simulink model "SixDOFSim"  (R2020b)
settings: Solver=VariableStepAuto  StartTime=0.0  StopTime=80  RelTol=1e-3
values from neighbouring files (symbols this model uses):
  A = sys_ol.A    [cost_condition_number.m]    (also in cost_coupling_control.m; cost_filter.m; coupling_control_scratch.m = sys.A; coupling_control_scratch2.m = sys.A)
  B = sys_ol.B    [cost_condition_number.m]    (also in cost_coupling_control.m; cost_filter.m; coupling_control_scratch.m = sys.B; coupling_control_scratch2.m = sys.B)
  C_tilde = zeros(size(C,1), size(A,1))    [SixDOFModel.m]    (also in cost_condition_number.m = struct_cond.C_tilde; cost_coupling_control.m = struct_cond.C_tilde; cost_filter.m = struct_cond.C_tilde; coupling_controller.m = T*C_resort)
  deltaX_init = Tx\deltaX_init    [SixDOFModel.m]    (also in coupling_controller_main.m = X_init-X_ap_simulink)
  eta_max = 15*pi/180    (= 0.261799387799)    [SixDOFModel.m]    (also in coupling_controller_main.m = 0.174532925199; load_messung_one_massmodel.m = 0.174532925199)
  eta_min = - 30*pi/180    (= -0.523598775598)    [SixDOFModel.m]    (also in coupling_controller_main.m = -0.436332312999; load_messung_one_massmodel.m = -0.436332312999)
  F = real(F)    [coupling_control_scratch.m]    (also in coupling_control_scratch2.m; coupling_controller.m = Kopt{end}; coupling_controller_main.m = -inv(C*(Ak\B)); coupling_controller_philipp.m = -inv(C*(Ak\B)))
  F_mod = F_ent(:,1:p/2)    [SixDOFModel.m]    (also in coupling_controller_main.m = F1*Q_mod; coupling_controller_philipp.m = F1*Q_mod; script_kein_theta_verk.m = F1*Q_mod)
  K_coupling = inv(Dstar)*compR    [SixDOFModel.m]    (also in coupling_controller_main.m = Kopt{1}; coupling_controller_philipp.m = Kopt{1}; script_kein_theta_verk.m = Kopt{1})
  latlon_init = [0;0]    [SixDOFModel.m]    (also in create_multi_model.m)
  m = i-1    [coupling_control_scratch.m]    (also in coupling_control_scratch2.m; defineABC.m = size(B_1,2) + size(B_2,2); implicit_linmod.m = length(U_ap); initializeParameters.m = 120000)
  noise_weight = [10 10 10 1 1 1 1 1 10 10 10 10 1 1 1 1 1 10]'    [SixDOFModel.m]
  P_e_init_1 = [0;0;-h_init_1]    [SixDOFModel.m]    (also in create_multi_model.m)
  P_e_init_2 = [0;0;-h_init_2]    [SixDOFModel.m]    (also in create_multi_model.m)
  q = X(5)    [nonlinear_6DOF.m]    (also in normieren.m = size (C,1))
  r = 5    [coupling_controller.m]    (also in coupling_controller_main.m = 100; coupling_controller_philipp.m = 200; nonlinear_6DOF.m = X(6); polgebiet.m = a2)
  sigmaf_max = 20*pi/180    (= 0.349065850399)    [SixDOFModel.m]    (also in coupling_controller_main.m; load_messung_one_massmodel.m)
  sigmaf_min = 0.5*pi/180    (= 0.00872664625997)    [SixDOFModel.m]    (also in coupling_controller_main.m; load_messung_one_massmodel.m)
  Tu = eye(size(B,2))    [SixDOFModel.m]    (also in normieren.m = zeros(p,p))
  Tx = eye(n)    [SixDOFModel.m]    (also in normieren.m = diag([200 15 50 0.1 0.1 0.1 45*pi/180 45*pi/180 10000 200 15)
  Ty = eye(size(C,1))    [SixDOFModel.m]    (also in normieren.m = zeros(q,q))
  U_ap = Tu\U_ap    [SixDOFModel.m]    (also in coupling_controller_main.m = AP(1,1).U_ap; create_multi_model.m = [U_ap_1;U_ap_2]; fsolve_trim.m = ap(11:14); trimValues.m = Z_ap(11:14))
  W_ap = W_ap(1:4)    [SixDOFModel.m]    (also in coupling_controller_philipp.m = (C*X_ap_simulink)')
  X_ap = [X_ap_1;X_ap_2]    [SixDOFModel.m]    (also in coupling_controller_main.m = AP(1,1).X_ap; create_multi_model.m; fsolve_trim.m = ap(1:10); trimValues.m = Z_ap(1:10))
  X_ap_simulink = Tx\X_ap_simulink    [SixDOFModel.m]    (also in coupling_controller_main.m = AP(1,1).X_ap_simulink; create_multi_model.m = [X_ap(1:8);X_ap(10);X_ap(11:18);X_ap(20)])
  X_init = Tx\X_init    [SixDOFModel.m]    (also in cost_coupling_control.m = struct_cond.X_init; cost_filter.m = struct_cond.X_init; coupling_controller_main.m = X_ap_simulink; create_multi_model.m = [X_init_1; X_init_2])
  xi_max = 25*pi/180    (= 0.436332312999)    [SixDOFModel.m]    (also in coupling_controller_main.m; load_messung_one_massmodel.m)
  xi_min = - xi_max    (= -0.436332312999)    [SixDOFModel.m]    (also in coupling_controller_main.m; load_messung_one_massmodel.m)
  zita_max = 30*pi/180    (= 0.523598775598)    [SixDOFModel.m]    (also in coupling_controller_main.m; load_messung_one_massmodel.m)
  zita_min = - zita_max    (= -0.523598775598)    [SixDOFModel.m]    (also in coupling_controller_main.m; load_messung_one_massmodel.m)
undefined symbols (not defined in the file or in its folder): Earth, globalParameters, Light, MIL, WGS84
libraries: aerolibfltsims x24, aerolibtransform2 x4, aerolibwind2 x4, simulink x3, shared6dof x1, aerolibanim x1
(part 3 of 3)

== matlab function SixDOFSim/6 DOF Non Linear Model Equations/MATLAB Function1 ==
  data: X input; dX output; U input; psi input; plane_selector input
function dX  = nonlinear_equations_simulink(X,U,psi,plane_selector)
%--------------States------------%
u = X(1);
v = X(2);
w = X(3);
p = X(4);
q = X(5);
r = X(6);
phi = X(7);
theta = X(8);
h = X(9);

%--------------Control------------%
eta = U(1);
sigmaf = U(2);
xi = U(3);
zita = U(4);

%--------------Constants------------%
%% Initialize
g = 9.81; %Gravity [m/s^2]
m = 120000; %Mass [kg]

%Refuel
m_fuel = 28000; %Mass of the fuel
time_refuel = 20; % Time to refuel in sec
start_time_refuel = 10; 
refuel = 0; %Without refuel = 1, with refuel = 0

% Modelling the atmosphere 
rho_const = 1.225; %Airdensity (simplification)
omega_e = 7.29211510*10^(-5); %Rotation Speed of earth [rad/s]
%omega_e = 0;
he = 6356752; %Earth radius [m]
Omega_e_tilde = vecToMat([0;0;omega_e]);

% Inertia and Paramethers of the plane
S = 260; % Flugfläche (wing platform area)
St = 64; %Aerea of the Tail [m^2] 
lt = 24.8; %Length to tail [m] (estimation)
l = 6.6; % generalized length [m]

%Moments of Inertia of Boeing 757-200 [kg(m^2]
% Ix = 10710000; % 
% Ixz = 0; 
% Iy = 14883800; 
% Iz = 25283271; 
% I = [Ix 0 Ixz;0 Iy 0;Ixz 0 Iz]; %Trägheitstensor
I = m*[40.07 0 2.09;0 64 0;2.09 0 99.92];
I_inv = inv(I);

b = 44.8; %Span [m] 
c = 6.6; % Wing Chord [m]

%Aerodynamical Positions
% P_centerGravity = [0.23*c;0;0];
% P_aerodynCenter = [0.12*c;0;0];
P_centerGravity = [0;0;0];
P_aerodynCenter = P_centerGravity;

%Motor and Thrust
%P_thrust = [0.23*c;0;0.1*c+1.9]; %Position of the motor [m] 
P_thrust = [0;0;1.9]; %Position of the motor [m] 
% P_thrust = P_centerGravity;
i_f = 0 ; %Direction of Thrus [rad];
F_max = m*g; %Warning - This is obviusly not the max thrust produced by the turbines. The max Turbine Force is considered on the maximum value of sigmaf

globalParameters.g = g;
globalParameters.m = m;
globalParameters.Omega_e_tilde = Omega_e_tilde;
globalParameters.rho_const = rho_const;
globalParameters.I = I;
globalParameters.I_inv = I_inv;
globalParameters.S = S;
globalParameters.St = St;
globalParameters.lt = lt;
globalParameters.b = b;
globalParameters.c = c;
globalParameters.l = l;
globalParameters.P_thrust =P_thrust;
globalParameters.P_centerGravity = P_centerGravity;
globalParameters.P_aerodynCenter = P_aerodynCenter;
globalParameters.i_f =i_f;
globalParameters.Fmax = F_max;
globalParameters.m_fuel = m_fuel;
globalParameters.time_refuel = time_refuel;
globalParameters.start_time_refuel = start_time_refuel;
globalParameters.refuel = refuel;

%%
T   = 288.15 - 0.0065*h;                    % Temperatur bei H
ps  = 101325*(T/288.15)^(g/1.86584);        % Statischer Luftdruck
rho = ps/(287.053*T);
if plane_selector == 1
    I = globalParameters.I ;
    S = globalParameters.S ;
    St = globalParameters.St ;
    lt = globalParameters.lt ;
    b = globalParameters.b ;
    c = globalParameters.c ;
    P_thrust = globalParameters.P_thrust ;
    P_centerGravity = globalParameters.P_centerGravity ;
    P_aerodynCenter = globalParameters.P_aerodynCenter ;
    i_f = globalParameters.i_f ;
    F_max = globalParameters.Fmax;
elseif plane_selector == 2
    I = globalParameters.I ;
    S = globalParameters.S ;
    St = globalParameters.St ;
    lt = globalParameters.lt ;
    b = globalParameters.b ;
    c = globalParameters.c ;
    P_thrust = globalParameters.P_thrust ;
    P_centerGravity = globalParameters.P_centerGravity ;
    P_aerodynCenter = globalParameters.P_aerodynCenter ;
    i_f = globalParameters.i_f ;
    F_max = globalParameters.Fmax;
end
    
% Airdynamical Coefficients
%CA0 = 1.104;
grad_alpha = 5.5;
alpha_L0 = -11.5*pi/180;
gradient_alpha_epsolon = 0.25;
gradient_CQ_Cbeta = -1.6;
gradientCQ_Czita = 0.24;
CW0 = 0.13;
kappa = 0.07;

% %--------------Variables------------%
% u = sqrt(vA^2*(1-sin(beta)^2)/(1+tan(alpha)^2));
% v = sin(beta)*vA;
% w = u*tan(alpha);
V = [u;v;w];
vA = sqrt(u^2+v^2+w^2);
alpha = atan(w/u);
beta = asin(v/vA);
gamma = theta - alpha;
dh = vA*sin(gamma);

q_d = 0.5*rho*vA^2; %Dynamic Preassure
Omega = [p;q;r];


%--------------Aerodynamical Coefficients------------%
%Forces Coefficients
CA_F = grad_alpha*(alpha - alpha_L0);
epsolon = gradient_alpha_epsolon*(alpha - alpha_L0); %Downwash [rad]
alpha_t = alpha - epsolon + eta +1.3*q*lt/vA; %Angle of Attack of the Tail [rad]
CA_H = 3.1*(St/S)*alpha_t; %Lift Coefficient of the Control Aereas (Elevator-Tail)
CA = CA_F + CA_H; %Total Lift Coefficient

CW = CW0 + kappa*(CA_F - 0.45)^2; %Drag Coefficient

CQ = gradient_CQ_Cbeta*beta + gradientCQ_Czita*zita; % Sideforce coefficient

%Moments Coefficients
N = [-1.4*beta;-0.59-3.1*(St*lt/(l*S))*(alpha-epsolon);(1-alpha*(180/(15*pi)))*beta]; %Static Moments Effects
Jakobi_CM_X = (l/vA)*[-11,    0,           5;
                      0,-4.03*St*lt^2/(S*l^2),0;
                      1.7,          0   , -11.5];
Jakobi_CM_U = [-0.6, 0, 0.22;
               0,    -3.1*St*lt/(S*l),0;
               0, 0, -0.63];      % Dependence of Control Variables
           
C_torque = N + Jakobi_CM_X*Omega + Jakobi_CM_U*[xi;eta;zita];
CL = C_torque(1);
CM = C_torque(2);
CN = C_torque(3);

%-------------- Forces and Moments ------------%
%Aerodynamics
A = q_d*S*CA; %Lift Force [N]
W = q_d*S*CW; %Air Resistance [N]
Q = q_d*S*CQ; %Transverse Force [N]

% EVTL VORZEICHEN VON BETA ÄNDERN
Tfa = coordTransfMatrix(alpha,2)*coordTransfMatrix(-beta,3); %Transformation Matrix Aerodynamics -> Körperfest

RA_a =[-W;Q;-A]; %Aerodynamical Force in Aerdodynamical Reference Frame
RA = Tfa*RA_a; %Aerodynamical Force in Body Reference Frame
QA_aerodynCenter = q_d*S*[b*CL*0.5;c*CM;b*CN*0.5]; %Torque on the aerodynamical Center
QA = QA_aerodynCenter + vecToMat(P_centerGravity- P_aerodynCenter)*RA; %Aerodynamical Force in Body Reference Frame


%Thrust
F_res = F_max*sigmaf; %Thrust Force Absolute Value
Rf = F_res*[cos(i_f);0;sin(i_f)]; %Thrust Force 
Qf = vecToMat(P_thrust - P_centerGravity)*Rf; %Thrust Moment

Q_total = Qf + QA; %Sum of external Moments in Body reference Frame [Nm]
R_total = RA + Rf; %Sum of external Forces in Body reference Frame [N]

%-------------- Equations of Motion ------------%
%Dynamic
Tfg =  coordTransfMatrix(phi,1)*coordTransfMatrix(theta,2)*coordTransfMatrix(psi,3); % Transformation Matrix goedetic --> body reference Frame
Tgf = Tfg.';%Transformation to North East Down
Omega_tilde = vecToMat(Omega);
dOmega = I_inv*(Q_total - Omega_tilde*I*Omega); %Derivative of Rotation Rate (body Reference Frame)

% ACHTUNG: Omega_e_tilde wurde in DGL für dV entfernt, da flache ERde
dV = R_total/m + Tfg*[0;0;g] - (Omega_tilde)*V; %Derivatitive of the Speed (body Reference Frame)
% dvA = (u*dV(1) + v*dV(2) + w*dV(3))/sqrt(u^2 + v^2 + w^2); %Derivative of the Approach Speed
% dalpha = (dV(3)*u - dV(1)*w)/(u^2 + u*w); %Derivative of Angle of Attack
% dbeta = (dV(2)*vA - dvA*V(2))/(vA*sqrt(vA^2 - V(2)^2)); %Derivative of Sideslip Angle

%Kinematics
dP_e = Tgf*V; % gilt nur für z-Komponente

% ACHTUNG: dh anders als im Buch ... Teg fehlt, sollte für dh keinen
% Unterschied machen
% dh = - dP_e(3); %Derivative of z-position (earth Reference Frame)

J = 1/cos(theta)*[cos(theta) sin(phi)*sin(theta) cos(phi)*sin(theta) ;0 cos(phi)*cos(theta) -sin(phi)*cos(theta);0 sin(phi) cos(phi)]; %Rotation rate matrix
dPhi = J*Omega; %Derivative of Euler Angles
dX = double([dV;dOmega;dPhi(1);dPhi(2);dh]);
end

== matlab function SixDOFSim/6 DOF Non Linear Model Equations/calc dpsi ==
  data: X input; dpsi output
function dpsi = fcn(X)
q = X(5);
r = X(6);
phi = X(7);
theta = X(8);
dpsi = (r*cos(phi))/cos(theta) + (q*sin(phi))/cos(theta);
end

== matlab function SixDOFSim/6 DOF Non Linear Model Equations/calc dpsi1 ==
  data: X input; dpsi output
function dpsi = fcn(X)
q = X(5);
r = X(6);
phi = X(7);
theta = X(8);
dpsi = (r*cos(phi))/cos(theta) + (q*sin(phi))/cos(theta);
end

== matlab function SixDOFSim/6 DOF Non Linear Model Equations/MATLAB Function2 ==
  data: X input; y output
function y = fcn(X)
u = X(1);
w = X(3);
theta = X(8);
y = theta - atan(w/u);
end

== matlab function SixDOFSim/6 DOF Model Boeing 757 200/MATLAB Function3 ==
  data: Phi input; DCM output
function DCM = getTfg(Phi)

DCM = coordTransfMatrix(Phi(1),1)*coordTransfMatrix(Phi(2),2)*coordTransfMatrix(Phi(3),3); % Transformation Matrix goedetic --> body reference Frame

== matlab function SixDOFSim/6 DOF Model Boeing 757 200/Rho/calc_rho ==
  data: h input; rho output; globalParameters parameter
function rho = fcn(h,globalParameters)
g = globalParameters.g;
T   = 288.15 - 0.0065*h;                    % Temperatur bei H
ps  = 101325*(T/288.15)^(g/1.86584);        % Statischer Luftdruck
rho = ps/(287.053*T);
end

== matlab function SixDOFSim/6 DOF Model Boeing 757 200/Geometrical Coefficients Plane 2/MATLAB Function ==
  data: V input; aero_angles output
function aero_angles = fcn(V)
u = V(1);
v = V(2);
w = V(3);
vA = sqrt(u^2+v^2+w^2);
alpha = atan(w/u);
beta = asin(v/vA);
aero_angles = [alpha beta];
end

== matlab function SixDOFSim/6 DOF Model Boeing 757 200/Wind1/abs(V) ==
  data: u input size=3; y output
function y = fcn(u)
y = sqrt(u(1)^2+u(2)^2+u(3)^2);
end

== matlab function SixDOFSim/6 DOF Model Boeing 757 200/Geometrical Coefficients Plane 2/calc_vA ==
  data: V_total input; vA output
function vA = fcn(V_total)

vA = sqrt(V_total(1)^2 + V_total(2)^2 + V_total(3)^2);

== matlab function SixDOFSim/6 DOF Model Boeing 757 200/Forces and Moments Plane 2/Aerodynamical Forces ==
  data: CA input; RA output size=3; CW input; CQ input; vA input; alpha input; beta input; rho input; globalParameters parameter
function RA = getAerodynForces(CA,CW,CQ,vA, alpha, beta, rho,globalParameters)

q_d = 0.5*vA^2*rho; %Dynamic Preassure
S = globalParameters.S ;

%Aerodynamics
A = q_d*S*CA; %Lift Force [N]
W = q_d*S*CW; %Air Resistance [N]
Q = q_d*S*CQ; %Transverse Force [N]

% EVTL VORZEICHEN VON BETA ÄNDERN
Tfa = coordTransfMatrix(alpha,2)*coordTransfMatrix(-beta,3); %Transformation Matrix Aerodynamics -> Körperfest

RA_a =[-W;Q;-A]; %Aerodynamical Force in Aerdodynamical Reference Frame
RA = Tfa*RA_a; %Aerodynamical Force in Body Reference Frame

== matlab function SixDOFSim/6 DOF Model Boeing 757 200/Forces and Moments Plane 2/Aerodynamical Torque ==
  data: RA input; CL input; QA output size=3; CM input; CN input; vA input; globalParameters parameter; rho input
function QA = getAerodynTorque(RA,CL,CM,CN, vA, globalParameters,rho)
%Aircraft Parameters
b = globalParameters.b;
c = globalParameters.c;
S = globalParameters.S;
P_centerGravity = globalParameters.P_centerGravity;
P_aerodynCenter = globalParameters.P_aerodynCenter;
q_d = 0.5*vA^2*rho; %Dynamic Preassure

QA_aerodynCenter = q_d*S*[b*CL*0.5;c*CM;b*CN*0.5]; %Torque on the aerodynamical Center
QA = QA_aerodynCenter + vecToMat(P_centerGravity- P_aerodynCenter)*RA; %Aerodynamical Force in Body Reference Frame

== matlab function SixDOFSim/6 DOF Model Boeing 757 200/Forces and Moments Plane 2/Thrust Force and Torque ==
  data: sigmaf input; Rf output; globalParameters parameter; Qf output
function [Rf,Qf] = thrust(sigmaf,globalParameters)
%Get Thrus Force Rf and Thrust Moment Qf
%sigmaf: Throttle Position [rad]
P_thrust =globalParameters.P_thrust;
i_f =globalParameters.i_f;
F_max = globalParameters.Fmax;
P_centerGravity = globalParameters.P_centerGravity;
%Thrust
F_res = F_max*sigmaf; %Thrust Force Absolute Value
Rf = F_res*[cos(i_f);0;sin(i_f)]; %Thrust Force 
Qf = vecToMat(P_thrust - P_centerGravity)*Rf; %Thrust Moment

== matlab function SixDOFSim/6 DOF Model Boeing 757 200/Motion model Plane 2/Dynamics/MATLAB Function ==
  data: Phi input; dV output; Omega input; V input; R_total input; Q_total input; globalParameters parameter; dOmega output; dPhi output
function [dV,dOmega,dPhi] = fcn(Phi, Omega, V, R_total, Q_total, globalParameters)
I_inv = globalParameters.I_inv;
I = globalParameters.I;
m = globalParameters.m;
g = globalParameters.g;
phi = Phi(1);
theta = Phi(2);
psi = Phi(3);
Tfg =  coordTransfMatrix(phi,1)*coordTransfMatrix(theta,2)*coordTransfMatrix(psi,3); % Transformation Matrix goedetic --> body reference Frame
Omega_tilde = vecToMat(Omega);
dOmega = I_inv*(Q_total - Omega_tilde*I*Omega); %Derivative of Rotation Rate (body Reference Frame)

% ACHTUNG: Omega_e_tilde wurde in DGL für dV entfernt, da flache ERde
dV = R_total/m + Tfg*[0;0;g] - (Omega_tilde)*V; %Derivatitive of the Speed (body Reference Frame)

J = 1/cos(theta)*[cos(theta) sin(phi)*sin(theta) cos(phi)*sin(theta) ;0 cos(phi)*cos(theta) -sin(phi)*cos(theta);0 sin(phi) cos(phi)]; %Rotation rate matrix
dPhi = J*Omega; %Derivative of Euler Angles
end

== matlab function SixDOFSim/6 DOF Model Boeing 757 200/Motion model Plane 2/Dynamics/Track and Aerodynamical Speed ==
  data: dxyh output; Phi input; V input; vk output; gamma output; chsi output
function [dxyh,vk,gamma,chsi] = getTrackAndAero(Phi,V)
%Get The Track Speed, the Approach Speed, the inclinational angle ,
%the Azimuth angle, the angle of attack and the Sliding angle from the
%Speed from the Translational Velocity. 
Tfg =  coordTransfMatrix(Phi(1),1)*coordTransfMatrix(Phi(2),2)*coordTransfMatrix(Phi(3),3); % Transformation Matrix goedetic --> body reference Frame
Tgf = Tfg';
Vk = Tgf*V; %Track Velocity
vk = sqrt(Vk(1)^2+Vk(2)^2+Vk(3)^2); %Track Speed [m/s]
gamma = -asin(Vk(3)/vk); %Inclination Angle [rad]
chsi = atan2(Vk(2),Vk(1));
dx = vk*cos(gamma)*cos(chsi);
dy = vk*cos(gamma)*sin(chsi);
dh = vk*sin(gamma);
dxyh = [dx; dy; dh];

== matlab function SixDOFSim/6 DOF Non Linear Model Equations/Visualisation Non Linear Model 1/Body to Earth Reference Frame  ==
  data: V input; Phi input; V_e output
function V_e = getEarthPosition(V,Phi)

Tfg = coordTransfMatrix(Phi(1),1)*coordTransfMatrix(Phi(2),2)*coordTransfMatrix(Phi(3),3); % Transformation Matrix goedetic --> body reference Frame
Tgf = Tfg';
V_e = Tgf*V;
V_e(3) =  V_e(3);

== matlab function SixDOFSim/6 DOF Model Boeing 757 200/Motion model Plane 2/Dynamics/Transformation of gravity in (Körperfestes System) ==
  data: Phi input; gravityAcceleration output; g parameter
function gravityAcceleration = Tfg(Phi,g)
G_geod = [0;0;g]; %Graviation vector in geodetic ref. Frame
Tfg = coordTransfMatrix(Phi(1),1)*coordTransfMatrix(Phi(2),2)*coordTransfMatrix(Phi(3),3); % Transformation Matrix goedetic --> body reference Frame
gravityAcceleration = Tfg*G_geod;

== matlab function SixDOFSim/6 DOF Model Boeing 757 200/Forces and Moments Plane 3/Aerodynamical Forces ==
  data: CA input; RA output size=3; CW input; CQ input; vA input; alpha input; beta input; rho input; globalParameters parameter
function RA = getAerodynForces(CA,CW,CQ,vA, alpha, beta, rho,globalParameters)

q_d = 0.5*vA^2*rho; %Dynamic Preassure
S = globalParameters.S ;

%Aerodynamics
A = q_d*S*CA; %Lift Force [N]
W = q_d*S*CW; %Air Resistance [N]
Q = q_d*S*CQ; %Transverse Force [N]

% EVTL VORZEICHEN VON BETA ÄNDERN
Tfa = coordTransfMatrix(alpha,2)*coordTransfMatrix(-beta,3); %Transformation Matrix Aerodynamics -> Körperfest

RA_a =[-W;Q;-A]; %Aerodynamical Force in Aerdodynamical Reference Frame
RA = Tfa*RA_a; %Aerodynamical Force in Body Reference Frame

== matlab function SixDOFSim/6 DOF Model Boeing 757 200/Forces and Moments Plane 3/Aerodynamical Torque ==
  data: RA input; CL input; QA output size=3; CM input; CN input; vA input; globalParameters parameter; rho input
function QA = getAerodynTorque(RA,CL,CM,CN, vA, globalParameters,rho)
%Aircraft Parameters
b = globalParameters.b;
c = globalParameters.c;
S = globalParameters.S;
P_centerGravity = globalParameters.P_centerGravity;
P_aerodynCenter = globalParameters.P_aerodynCenter;
q_d = 0.5*vA^2*rho; %Dynamic Preassure

QA_aerodynCenter = q_d*S*[b*CL*0.5;c*CM;b*CN*0.5]; %Torque on the aerodynamical Center
QA = QA_aerodynCenter + vecToMat(P_centerGravity- P_aerodynCenter)*RA; %Aerodynamical Force in Body Reference Frame

== matlab function SixDOFSim/6 DOF Model Boeing 757 200/Forces and Moments Plane 3/Thrust Force and Torque ==
  data: sigmaf input; Rf output; globalParameters parameter; Qf output
function [Rf,Qf] = thrust(sigmaf,globalParameters)
%Get Thrus Force Rf and Thrust Moment Qf
%sigmaf: Throttle Position [rad]
P_thrust =globalParameters.P_thrust;
i_f =globalParameters.i_f;
F_max = globalParameters.Fmax;
P_centerGravity = globalParameters.P_centerGravity;
%Thrust
F_res = F_max*sigmaf; %Thrust Force Absolute Value
Rf = F_res*[cos(i_f);0;sin(i_f)]; %Thrust Force 
Qf = vecToMat(P_thrust - P_centerGravity)*Rf; %Thrust Moment

== matlab function SixDOFSim/6 DOF Model Boeing 757 200/Geometrical Coefficients Plane 3/Geometrie Rotational Coefficients ==
  data: vA input; alpha input; beta input; Omega input; eta input; zita input; globalParameters parameter; xi input; CL output; CM output; CN output
function [CL,CM,CN] = torqueGeometricCoefficient(vA, alpha,beta,Omega,eta,zita, globalParameters,xi)
%eta = Höheruderwinkel (elevator) [rad]
%zita = Seitenruderwinkel (ruder) [rad]
%xi = Querruderwinkel (Airlon) [rad]
%Global Parameters
lt = globalParameters.lt;
l = globalParameters.l;
S = globalParameters.S;
St = globalParameters.St;

%Constants Coefficients
alpha_L0 = -11.5*pi/180;
gradient_alpha_epsolon = 0.25;
epsolon = gradient_alpha_epsolon*(alpha - alpha_L0); %Downwash [rad]

%Moments Coefficients
N = [-1.4*beta;-0.59-3.1*(St*lt/(l*S))*(alpha-epsolon);(1-alpha*(180/(15*pi)))*beta]; %Static Moments Effects
Jakobi_CM_X = (l/vA)*[-11,    0,           5;
                      0,-4.03*St*lt^2/(S*l^2),0;
                      1.7,          0   , -11.5];
Jakobi_CM_U = [-0.6, 0, 0.22;
               0,    -3.1*St*lt/(S*l),0;
               0, 0, -0.63];      % Dependence of Control Variables
           
C_torque = N + Jakobi_CM_X*Omega + Jakobi_CM_U*[xi;eta;zita];
CL = C_torque(1);
CM = C_torque(2);
CN = C_torque(3);

== matlab function SixDOFSim/6 DOF Model Boeing 757 200/Geometrical Coefficients Plane 3/Geometry Translational Coefficients ==
  data: vA input; alpha input; beta input; CA output; Omega input; globalParameters parameter; CW output; CQ output; eta input; zita input
function [CA,CW,CQ] = forceGeometryCoefficients(vA, alpha,beta,Omega,globalParameters,eta,zita)
%eta = Höheruderwinkel (elevator) [rad]
%zita = Seitenruderwinkel (ruder) [rad]
%Global Parameters
lt = globalParameters.lt;
S = globalParameters.S;
St = globalParameters.St;

% Rotration rates [rad/s]
q = Omega(2); %Nickrate (Pitch Rate)

%Constants Coefficients
grad_alpha = 5.5;
alpha_L0 = -11.5*pi/180;
gradient_alpha_epsolon = 0.25;
gradient_CQ_Cbeta = -1.6;
gradientCQ_Czita = 0.24;
CW0 = 0.13;
kappa = 0.07;

%Forces Coefficients
CA_F = grad_alpha*(alpha - alpha_L0);
epsolon = gradient_alpha_epsolon*(alpha - alpha_L0); %Downwash [rad]
alpha_t = alpha - epsolon + eta +1.3*q*lt/vA; %Angle of Attack of the Tail [rad]
CA_H = 3.1*(St/S)*alpha_t; %Lift Coefficient of the Control Aereas (Elevator-Tail)
CA = CA_F + CA_H; %Total Lift Coefficient
CW = CW0 + kappa*(CA_F - 0.45)^2; %Drag Coefficient
CQ = gradient_CQ_Cbeta*beta + gradientCQ_Czita*zita; % Sideforce coefficient

== matlab function SixDOFSim/6 DOF Model Boeing 757 200/Geometrical Coefficients Plane 3/MATLAB Function ==
  data: V input; aero_angles output
function aero_angles = fcn(V)
u = V(1);
v = V(2);
w = V(3);
vA = sqrt(u^2+v^2+w^2);
alpha = atan(w/u);
beta = asin(v/vA);
aero_angles = [alpha beta];

== matlab function SixDOFSim/6 DOF Non Linear Model Equations/Visualisation Non Linear Model 1/MATLAB Function ==
  data: V input; vA output; alpha output; beta output
function [vA,alpha,beta] = getAerodynamical(V)
u = V(1);
v = V(2);
w = V(3);
vA = sqrt(u^2+v^2+w^2);
alpha = atan2(w,u);
beta = asin(v/vA);

== matlab function SixDOFSim/6 DOF Model Boeing 757 200/Geometrical Coefficients Plane 3/calc_vA ==
  data: V_total input; vA output
function vA = fcn(V_total)

vA = sqrt(V_total(1)^2 + V_total(2)^2 + V_total(3)^2);

== matlab function SixDOFSim/6 DOF Model Boeing 757 200/MATLAB Function4 ==
  data: Phi input; DCM output
function DCM = getTfg(Phi)

DCM = coordTransfMatrix(Phi(1),1)*coordTransfMatrix(Phi(2),2)*coordTransfMatrix(Phi(3),3); % Transformation Matrix goedetic --> body reference Frame

== matlab function SixDOFSim/6 DOF Model Boeing 757 200/Motion model Plain3/Dynamics/MATLAB Function ==
  data: Phi input; dV output; Omega input; V input; R_total input; Q_total input; globalParameters parameter; dOmega output; dPhi output
function [dV, dOmega, dPhi] = fcn(Phi, Omega, V, R_total, Q_total, globalParameters)
I_inv = globalParameters.I_inv;
I = globalParameters.I;
m = globalParameters.m;
g = globalParameters.g;
phi = Phi(1);
theta = Phi(2);
psi = Phi(3);
Tfg =  coordTransfMatrix(phi,1)*coordTransfMatrix(theta,2)*coordTransfMatrix(psi,3); % Transformation Matrix goedetic --> body reference Frame
Omega_tilde = vecToMat(Omega);
dOmega = I_inv*(Q_total - Omega_tilde*I*Omega); %Derivative of Rotation Rate (body Reference Frame)

% ACHTUNG: Omega_e_tilde wurde in DGL für dV entfernt, da flache ERde
dV = R_total/m + Tfg*[0;0;g] - (Omega_tilde)*V; %Derivatitive of the Speed (body Reference Frame)

J = 1/cos(theta)*[cos(theta) sin(phi)*sin(theta) cos(phi)*sin(theta) ;0 cos(phi)*cos(theta) -sin(phi)*cos(theta);0 sin(phi) cos(phi)]; %Rotation rate matrix
dPhi = J*Omega; %Derivative of Euler Angles
end

== matlab function SixDOFSim/6 DOF Model Boeing 757 200/Motion model Plain3/Dynamics/Track and Aerodynamical Speed ==
  data: dxyh output; Phi input size=3; V input; vk output; gamma output; chsi output
function [dxyh,vk,gamma,chsi] = getTrackAndAero(Phi,V)
%Get The Track Speed, the Approach Speed, the inclinational angle ,
%the Azimuth angle, the angle of attack and the Sliding angle from the
%Speed from the Translational Velocity. 
Tfg = coordTransfMatrix(Phi(1),1)*coordTransfMatrix(Phi(2),2)*coordTransfMatrix(Phi(3),3); % Transformation Matrix goedetic --> body reference Frame
Tgf = Tfg';
Vk = Tgf*V; %Track Velocity
vk = sqrt(Vk(1)^2+Vk(2)^2+Vk(3)^2); %Track Speed [m/s]
gamma = -asin(Vk(3)/vk); %Inclination Angle [rad]
chsi = atan2(Vk(2),Vk(1));
dx = vk*cos(gamma)*cos(chsi);
dy = vk*cos(gamma)*sin(chsi);
dh = vk*sin(gamma);
dxyh = [dx; dy; dh];

== matlab function SixDOFSim/6 DOF Model Boeing 757 200/Motion model Plain3/Dynamics/Transformation of gravity in (Körperfestes System) ==
  data: Phi input; gravityAcceleration output; g parameter
function gravityAcceleration = Tfg(Phi,g)
G_geod = [0;0;g]; %Graviation vector in geodetic ref. Frame
Tfg = coordTransfMatrix(Phi(1),1)*coordTransfMatrix(Phi(2),2)*coordTransfMatrix(Phi(3),3); % Transformation Matrix goedetic --> body reference Frame
gravityAcceleration = Tfg*G_geod;

== matlab function SixDOFSim/6 DOF Model Boeing 757 200/Rho1/calc_rho ==
  data: h input; rho output; globalParameters parameter
function rho = fcn(h,globalParameters)
g = globalParameters.g;
T   = 288.15 - 0.0065*h;                    % Temperatur bei H
ps  = 101325*(T/288.15)^(g/1.86584);        % Statischer Luftdruck
rho = ps/(287.053*T);
end

== matlab function SixDOFSim/6 DOF Linear/Visualisation Non Linear Model Plain 2/Body to Earth Reference Frame  ==
  data: V input; Phi input; V_e output
function V_e = getEarthPosition(V,Phi)

Tfg = coordTransfMatrix(Phi(1),1)*coordTransfMatrix(Phi(2),2)*coordTransfMatrix(Phi(3),3); % Transformation Matrix goedetic --> body reference Frame
Tgf = Tfg';
V_e = Tgf*V;
V_e(3) =  V_e(3);

== matlab function SixDOFSim/6 DOF Linear/Visualisation Non Linear Model Plain 2/MATLAB Function ==
  data: V input; vA output; alpha output; beta output
function [vA,alpha,beta] = getAerodynamical(V)
u = V(1);
v = V(2);
w = V(3);
vA = sqrt(u^2+v^2+w^2);
alpha = atan2(w,u);
beta = asin(v/vA);

== matlab function SixDOFSim/6 DOF Model Boeing 757 200/Geometrical Coefficients Plane 2/Geometrie Rotational Coefficients ==
  data: vA input; alpha input; beta input; Omega input; eta input; zita input; globalParameters parameter; xi input; CL output; CM output; CN output
function [CL,CM,CN] = torqueGeometricCoefficient(vA, alpha,beta,Omega,eta,zita, globalParameters,xi)
%eta = Höheruderwinkel (elevator) [rad]
%zita = Seitenruderwinkel (ruder) [rad]
%xi = Querruderwinkel (Airlon) [rad]
%Global Parameters
lt = globalParameters.lt;
l = globalParameters.l;
S = globalParameters.S;
St = globalParameters.St;

%Constants Coefficients
alpha_L0 = -11.5*pi/180;
gradient_alpha_epsolon = 0.25;
epsolon = gradient_alpha_epsolon*(alpha - alpha_L0); %Downwash [rad]

%Moments Coefficients
N = [-1.4*beta;-0.59-3.1*(St*lt/(l*S))*(alpha-epsolon);(1-alpha*(180/(15*pi)))*beta]; %Static Moments Effects
Jakobi_CM_X = (l/vA)*[-11,    0,           5;
                      0,-4.03*St*lt^2/(S*l^2),0;
                      1.7,          0   , -11.5];
Jakobi_CM_U = [-0.6, 0, 0.22;
               0,    -3.1*St*lt/(S*l),0;
               0, 0, -0.63];      % Dependence of Control Variables
           
C_torque = N + Jakobi_CM_X*Omega + Jakobi_CM_U*[xi;eta;zita];
CL = C_torque(1);
CM = C_torque(2);
CN = C_torque(3);

== matlab function SixDOFSim/6 DOF Model Boeing 757 200/Wind/abs(V) ==
  data: u input size=3; y output
function y = fcn(u)
y = sqrt(u(1)^2+u(2)^2+u(3)^2);
end

== matlab function SixDOFSim/6 DOF Model Boeing 757 200/Geometrical Coefficients Plane 2/Geometry Translational Coefficients ==
  data: vA input; alpha input; beta input; CA output; Omega input; globalParameters parameter; CW output; CQ output; eta input; zita input
function [CA,CW,CQ] = forceGeometryCoefficients(vA, alpha,beta,Omega,globalParameters,eta,zita)
%eta = Höheruderwinkel (elevator) [rad]
%zita = Seitenruderwinkel (ruder) [rad]
%Global Parameters
lt = globalParameters.lt;
S = globalParameters.S;
St = globalParameters.St;

% Rotration rates [rad/s]
q = Omega(2); %Nickrate (Pitch Rate)

%Constants Coefficients
grad_alpha = 5.5;
alpha_L0 = -11.5*pi/180;
gradient_alpha_epsolon = 0.25;
gradient_CQ_Cbeta = -1.6;
gradientCQ_Czita = 0.24;
CW0 = 0.13;
kappa = 0.07;

%Forces Coefficients
CA_F = grad_alpha*(alpha - alpha_L0);
epsolon = gradient_alpha_epsolon*(alpha - alpha_L0); %Downwash [rad]
alpha_t = alpha - epsolon + eta +1.3*q*lt/vA; %Angle of Attack of the Tail [rad]
CA_H = 3.1*(St/S)*alpha_t; %Lift Coefficient of the Control Aereas (Elevator-Tail)
CA = CA_F + CA_H; %Total Lift Coefficient
CW = CW0 + kappa*(CA_F - 0.45)^2; %Drag Coefficient
CQ = gradient_CQ_Cbeta*beta + gradientCQ_Czita*zita; % Sideforce coefficient

== matlab function SixDOFSim/6 DOF Non Linear Model Equations/Visualisation Non Linear Model 2/Body to Earth Reference Frame  ==
  data: V input; Phi input; V_e output
function V_e = getEarthPosition(V,Phi)

Tfg = coordTransfMatrix(Phi(1),1)*coordTransfMatrix(Phi(2),2)*coordTransfMatrix(Phi(3),3); % Transformation Matrix goedetic --> body reference Frame
Tgf = Tfg';
V_e = Tgf*V;
V_e(3) =  V_e(3);
